simulink model "testetm"  (R2021a)
settings: Solver=ode4  StartTime=0.0  StopTime=10.0  FixedStep=0.01  RelTol=1e-3
libraries: simulink x1
settings Model: Creator=ponyc  LastModifiedBy=ponyc

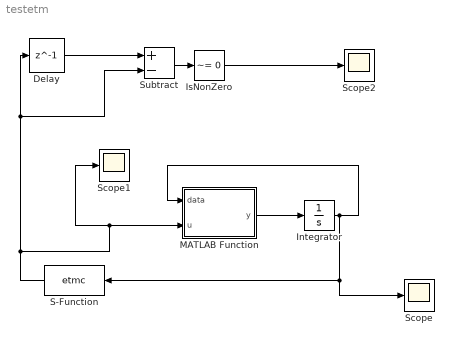
== system testetm ==
  Delay : Delay  DelayLength=1
  Integrator : Integrator  InitialCondition=10
  IsNonZero : simulink/Logic and Bit Operations/Compare To Zero  relop=~=  OutDataTypeStr=boolean
  MATLAB Function : MATLAB Function  TreatAsAtomicUnit=on
  S-Function : S-Function  FunctionName=etmc  SFunctionDeploymentMode=off  EnableBusSupport=off
  Scope : Scope
  Scope1 : Scope
  Scope2 : Scope
  Subtract : Sum  Inputs=+-
  wires:
  MATLAB Function/1(y) -> Integrator/1
  Integrator/1 -> Scope/1, S-Function/1, MATLAB Function/1(data)
  S-Function/1 -> Subtract/2, Delay/1, Scope1/1, MATLAB Function/2(u)
  Delay/1 -> Subtract/1
  IsNonZero/1 -> Scope2/1
  Subtract/1 -> IsNonZero/1

== matlab function testetm/MATLAB Function ==
  data: data input; u input; y output
function y = fcn(data, u)

y =data^2+ u;
